simulink model "r_controller_system_integrated"  (R2024a)
settings: Solver=ode23tb  StartTime=0.0  StopTime=0.1  FixedStep=1e-5  MaxStep=1e-05  RelTol=1e-3
libraries: simulink x1
settings Model: Creator=PME406_01  LastModifiedBy=PME406_01

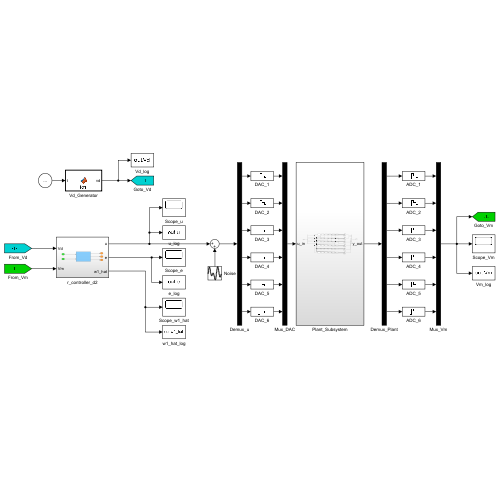
[thumbnail: Simulink's stored preview of the top-level diagram]
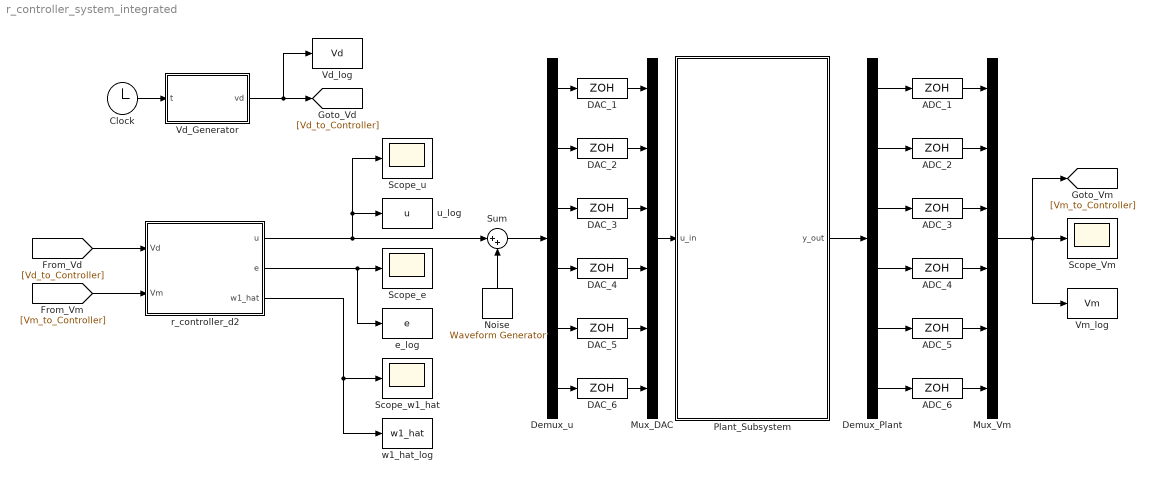
== system r_controller_system_integrated ==
  ADC_{1..6} (6 alike) : ZeroOrderHold  SampleTime=1e-05
  Clock : Clock
  DAC_{1..6} (6 alike) : ZeroOrderHold  SampleTime=1e-05
  Demux_Plant : Demux  Outputs=6
  Demux_u : Demux  Outputs=6
  Mux_DAC : Mux  Inputs=6
  Mux_Vm : Mux  Inputs=6
  Noise : simulink/Sources/Waveform Generator  OutMin=[]  OutMax=[]  OutDataTypeStr=double  SelectedSignal=1  BlockNames=MultiportSwitch_e3df3653d217406  SampleTime=0.1
  Plant_Subsystem : Subsystem
  Scope_Vm : Scope
  Scope_e : Scope
  Scope_u : Scope
  Scope_w1_hat : Scope
  Sum : Sum  Inputs=|++
  Vd_Generator : MATLAB Function  TreatAsAtomicUnit=on
  Vd_log : ToWorkspace  VariableName=Vd  SampleTime=-1
      settings: Save2DSignal=2-D array (concatenate along first dimension)
  Vm_log : ToWorkspace  VariableName=Vm  SampleTime=-1
      settings: Save2DSignal=2-D array (concatenate along first dimension)
  e_log : ToWorkspace  VariableName=e  SampleTime=-1
      settings: Save2DSignal=2-D array (concatenate along first dimension)
  r_controller_d2 : Subsystem
  u_log : ToWorkspace  VariableName=u  SampleTime=-1
      settings: Save2DSignal=2-D array (concatenate along first dimension)
  w1_hat_log : ToWorkspace  VariableName=w1_hat  SampleTime=-1
      settings: Save2DSignal=2-D array (concatenate along first dimension)
  wires:
  Vd_Generator/1(vd) -> Vd_log/1, [Vd_to_Controller]
  Clock/1 -> Vd_Generator/1(t)
  Mux_Vm/1 -> Vm_log/1, Scope_Vm/1, [Vm_to_Controller]
  ADC_6/1 -> Mux_Vm/6
  Demux_u/5 -> DAC_5/1
  DAC_4/1 -> Mux_DAC/4
  ADC_2/1 -> Mux_Vm/2
  Demux_u/6 -> DAC_6/1
  Sum/1 -> Demux_u/1
  ADC_4/1 -> Mux_Vm/4
  DAC_3/1 -> Mux_DAC/3
  r_controller_d2/1(u) -> Scope_u/1, u_log/1, Sum/1
  DAC_1/1 -> Mux_DAC/1
  DAC_2/1 -> Mux_DAC/2
  Demux_u/1 -> DAC_1/1
  Plant_Subsystem/1(y_out) -> Demux_Plant/1
  Demux_Plant/2 -> ADC_2/1
  Demux_Plant/5 -> ADC_5/1
  Noise/1 -> Sum/2
  ADC_3/1 -> Mux_Vm/3
  ADC_1/1 -> Mux_Vm/1
  r_controller_d2/3(w1_hat) -> w1_hat_log/1, Scope_w1_hat/1
  [Vm_to_Controller] -> r_controller_d2/2(Vm)
  Demux_Plant/4 -> ADC_4/1
  DAC_5/1 -> Mux_DAC/5
  Demux_u/3 -> DAC_3/1
  Demux_Plant/3 -> ADC_3/1
  Demux_Plant/1 -> ADC_1/1
  DAC_6/1 -> Mux_DAC/6
  Demux_u/4 -> DAC_4/1
  Mux_DAC/1 -> Plant_Subsystem/1(u_in)
  r_controller_d2/2(e) -> e_log/1, Scope_e/1
  Demux_u/2 -> DAC_2/1
  ADC_5/1 -> Mux_Vm/5
  Demux_Plant/6 -> ADC_6/1
  [Vd_to_Controller] -> r_controller_d2/1(Vd)

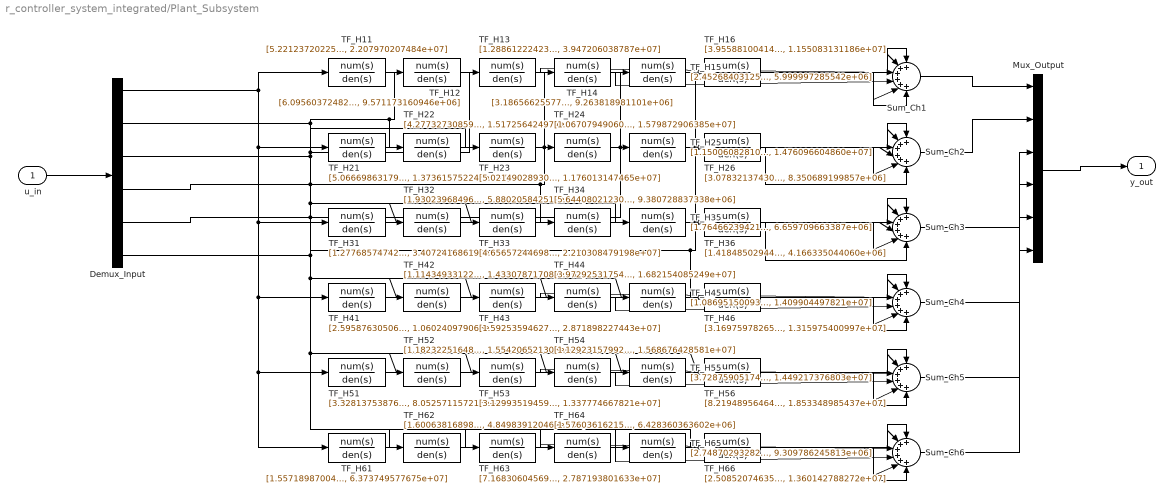
== system r_controller_system_integrated/Plant_Subsystem ==
  u_in : Inport
  Demux_Input : Demux  Outputs=6
  Mux_Output : Mux  Inputs=6
  Sum_Ch{1..6} (6 alike) : Sum  Inputs=++++++
  TF_H11 : TransferFcn  Numerator=[5.221237202258e+06]  Denominator=[1, 1.125476429798e+04, 2.207970207484e+07]
  TF_H12 : TransferFcn  Numerator=[6.095603724823e+04]  Denominator=[1, 1.615096196557e+03, 9.571173160946e+06]
  TF_H13 : TransferFcn  Numerator=[1.288612224236e+06]  Denominator=[1, 1.231137597589e+04, 3.947206038787e+07]
  TF_H14 : TransferFcn  Numerator=[3.186566255776e+05]  Denominator=[1, 7.765927137710e+03, 9.263818981101e+06]
  TF_H15 : TransferFcn  Numerator=[2.452684031253e+05]  Denominator=[1, 5.746401647961e+03, 5.999997285542e+06]
  TF_H16 : TransferFcn  Numerator=[3.955881004140e+05]  Denominator=[1, 3.580306515557e+03, 1.155083131186e+07]
  TF_H21 : TransferFcn  Numerator=[5.066698631790e+04]  Denominator=[1, 1.108261849372e+03, 1.373615752245e+07]
  TF_H22 : TransferFcn  Numerator=[4.277327308593e+06]  Denominator=[1, 1.003268373777e+04, 1.517256424974e+07]
  TF_H23 : TransferFcn  Numerator=[5.021490289304e+05]  Denominator=[1, 8.810895080316e+03, 1.176013147465e+07]
  TF_H24 : TransferFcn  Numerator=[1.067079490600e+06]  Denominator=[1, 1.135112820448e+04, 1.579872906385e+07]
  TF_H25 : TransferFcn  Numerator=[1.150060828107e+06]  Denominator=[1, 1.065992916636e+04, 1.476096604860e+07]
  TF_H26 : TransferFcn  Numerator=[3.078321374306e+05]  Denominator=[1, 6.847783968129e+03, 8.350689199857e+06]
  TF_H31 : TransferFcn  Numerator=[1.277685747428e+06]  Denominator=[1, 1.368269686933e+04, 3.407241686199e+07]
  TF_H32 : TransferFcn  Numerator=[1.930239684968e+05]  Denominator=[1, 4.560870597302e+03, 5.880205842512e+06]
  TF_H33 : TransferFcn  Numerator=[4.656572446985e+06]  Denominator=[1, 9.513164457161e+03, 2.210308479198e+07]
  TF_H34 : TransferFcn  Numerator=[5.644080212304e+04]  Denominator=[1, 1.954878812118e+03, 9.380728837338e+06]
  TF_H35 : TransferFcn  Numerator=[1.764662394212e+05]  Denominator=[1, 5.122349981324e+03, 6.659709663387e+06]
  TF_H36 : TransferFcn  Numerator=[1.418485029440e+05]  Denominator=[1, 1.438504147902e+03, 4.166335044060e+06]
  TF_H41 : TransferFcn  Numerator=[2.595876305066e+05]  Denominator=[1, 7.070165651413e+03, 1.060240979066e+07]
  TF_H42 : TransferFcn  Numerator=[1.114349331223e+06]  Denominator=[1, 9.846928206402e+03, 1.433078717084e+07]
  TF_H43 : TransferFcn  Numerator=[1.592535946272e+05]  Denominator=[1, 2.790294019501e+03, 2.871898227443e+07]
  TF_H44 : TransferFcn  Numerator=[3.972925317547e+06]  Denominator=[1, 1.159715140811e+04, 1.682154085249e+07]
  TF_H45 : TransferFcn  Numerator=[1.086951500933e+06]  Denominator=[1, 1.075231371220e+04, 1.409904497821e+07]
  TF_H46 : TransferFcn  Numerator=[3.169759782656e+05]  Denominator=[1, 8.067558736035e+03, 1.315975400997e+07]
  TF_H51 : TransferFcn  Numerator=[3.328137538766e+05]  Denominator=[1, 7.227274813518e+03, 8.052571157216e+06]
  TF_H52 : TransferFcn  Numerator=[1.182322516481e+06]  Denominator=[1, 1.030784744910e+04, 1.554206521303e+07]
  TF_H53 : TransferFcn  Numerator=[3.129935194599e+05]  Denominator=[1, 7.870328655037e+03, 1.337774667821e+07]
  TF_H54 : TransferFcn  Numerator=[1.129231579925e+06]  Denominator=[1, 1.104821595243e+04, 1.568676428581e+07]
  TF_H55 : TransferFcn  Numerator=[3.728759051745e+06]  Denominator=[1, 1.050075182774e+04, 1.449217376803e+07]
  TF_H56 : TransferFcn  Numerator=[8.219489564647e+04]  Denominator=[1, 1.407969854523e+03, 1.853348985437e+07]
  TF_H61 : TransferFcn  Numerator=[1.557189870041e+06]  Denominator=[1, 2.234640585923e+04, 6.373749577675e+07]
  TF_H62 : TransferFcn  Numerator=[1.600638168987e+05]  Denominator=[1, 3.864055922471e+03, 4.849839120469e+06]
  TF_H63 : TransferFcn  Numerator=[7.168306045699e+05]  Denominator=[1, 9.251556589809e+03, 2.787193801633e+07]
  TF_H64 : TransferFcn  Numerator=[1.576036162155e+05]  Denominator=[1, 4.743270970318e+03, 6.428360363602e+06]
  TF_H65 : TransferFcn  Numerator=[2.748702932822e+04]  Denominator=[1, 4.876033357949e+02, 9.309786245813e+06]
  TF_H66 : TransferFcn  Numerator=[2.508520746356e+06]  Denominator=[1, 5.985310903650e+03, 1.360142788272e+07]
  y_out : Outport
  wires:
  u_in/1 -> Demux_Input/1
  Demux_Input/1 -> TF_H11/1, TF_H51/1, TF_H61/1, TF_H41/1, TF_H31/1, TF_H21/1
  TF_H11/1 -> Sum_Ch1/1
  Demux_Input/2 -> TF_H12/1, TF_H22/1, TF_H52/1, TF_H62/1, TF_H42/1, TF_H32/1
  TF_H12/1 -> Sum_Ch1/2
  Demux_Input/3 -> TF_H13/1, TF_H23/1, TF_H53/1, TF_H63/1, TF_H43/1, TF_H33/1
  TF_H13/1 -> Sum_Ch1/3
  Demux_Input/4 -> TF_H54/1, TF_H64/1, TF_H44/1, TF_H14/1, TF_H24/1, TF_H34/1
  TF_H14/1 -> Sum_Ch1/4
  Demux_Input/5 -> TF_H55/1, TF_H65/1, TF_H45/1, TF_H15/1, TF_H25/1, TF_H35/1
  TF_H15/1 -> Sum_Ch1/5
  Demux_Input/6 -> TF_H16/1, TF_H26/1, TF_H36/1, TF_H46/1, TF_H56/1, TF_H66/1
  TF_H16/1 -> Sum_Ch1/6
  TF_H21/1 -> Sum_Ch2/1
  TF_H22/1 -> Sum_Ch2/2
  TF_H23/1 -> Sum_Ch2/3
  TF_H24/1 -> Sum_Ch2/4
  TF_H25/1 -> Sum_Ch2/5
  TF_H26/1 -> Sum_Ch2/6
  TF_H31/1 -> Sum_Ch3/1
  TF_H32/1 -> Sum_Ch3/2
  TF_H33/1 -> Sum_Ch3/3
  TF_H34/1 -> Sum_Ch3/4
  TF_H35/1 -> Sum_Ch3/5
  TF_H36/1 -> Sum_Ch3/6
  TF_H41/1 -> Sum_Ch4/1
  TF_H42/1 -> Sum_Ch4/2
  TF_H43/1 -> Sum_Ch4/3
  TF_H44/1 -> Sum_Ch4/4
  TF_H45/1 -> Sum_Ch4/5
  TF_H46/1 -> Sum_Ch4/6
  TF_H51/1 -> Sum_Ch5/1
  TF_H52/1 -> Sum_Ch5/2
  TF_H53/1 -> Sum_Ch5/3
  TF_H54/1 -> Sum_Ch5/4
  TF_H55/1 -> Sum_Ch5/5
  TF_H56/1 -> Sum_Ch5/6
  TF_H61/1 -> Sum_Ch6/1
  TF_H62/1 -> Sum_Ch6/2
  TF_H63/1 -> Sum_Ch6/3
  TF_H64/1 -> Sum_Ch6/4
  TF_H65/1 -> Sum_Ch6/5
  TF_H66/1 -> Sum_Ch6/6
  Sum_Ch1/1 -> Mux_Output/1
  Sum_Ch2/1 -> Mux_Output/2
  Sum_Ch3/1 -> Mux_Output/3
  Sum_Ch4/1 -> Mux_Output/4
  Sum_Ch5/1 -> Mux_Output/5
  Sum_Ch6/1 -> Mux_Output/6
  Mux_Output/1 -> y_out/1

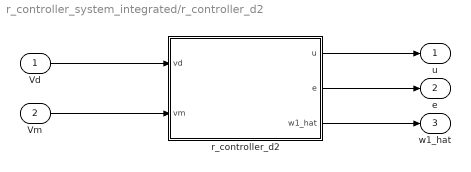
== system r_controller_system_integrated/r_controller_d2 ==
  Vd : Inport
  Vm : Inport  Port=2
  r_controller_d2 : MATLAB Function  TreatAsAtomicUnit=on
  u : Outport
  e : Outport  Port=2
  w1_hat : Outport  Port=3
  wires:
  r_controller_d2/3(w1_hat) -> w1_hat/1
  r_controller_d2/2(e) -> e/1
  Vm/1 -> r_controller_d2/2(vm)
  Vd/1 -> r_controller_d2/1(vd)
  r_controller_d2/1(u) -> u/1

== matlab function r_controller_system_integrated/r_controller_d2/r_controller_d2 ==
  settings: updateMethod=DISCRETE  sampleTime=1e-5
  data: vd input size=6; u output size=6; vm input size=6; e output size=6; w1_hat output size=6
function [u, e, w1_hat] = r_controller_function_d2(vd, vm)
    % R Controller with d=2 Preview (Flux_Control_R_newmodel.pdf Page 1)
    %
    % 完全平移時序方案：所有估測器公式從 k+1 平移到 k
    % 輸入：
    %   vd - 參考電壓向量 [6×1]（需要外部提供 3 步 preview）
    %   vm - 測量電壓向量 [6×1]
    % 輸出：
    %   u      - 控制輸入向量 [6×1]
    %   e      - 追蹤誤差向量 [6×1]（定義為 δv[k]）
    %   w1_hat - 干擾估測向量 [6×1]（用於監測干擾大小）
    %
    % Author: Claude Code
    % Date: 2025-10-16
    % Reference: Flux_Control_R_newmodel.pdf Page 1

    % ═══════════════════════════════════════════════════════════════════
    %                    SECTION 1: 參數定義
    % ═══════════════════════════════════════════════════════════════════

    % --- 系統模型參數 (from H(z^-1)) ---
    k_o = 5.6695e-4;              % k_o from H(z^-1)
    b = 0.9782;                   % b from H(z^-1)
    a1 = 1.934848;                % a1
    a2 = -0.935970;               % a2

    % --- B 矩陣 (6×6) ---
    B = [0.2365  -0.0064  -0.0327  -0.0344  -0.0408  -0.0343;
        -0.0037   0.2818  -0.0427  -0.0675  -0.0779  -0.0368;
        -0.0375  -0.0328   0.2108  -0.0060  -0.0265  -0.0341;
        -0.0245  -0.0777  -0.0056   0.2361  -0.0770  -0.0241;
        -0.0413  -0.0760  -0.0234  -0.0720   0.2572  -0.0045;
        -0.0244  -0.0330  -0.0257  -0.0245  -0.0030   0.1845];

    % --- B 反矩陣 ---
    B_inv = inv(B);

    % --- 控制參數 ---
    lambda_c = 0.8179;            % λc - 控制器特徵值
    lambda_e = 0.3659;            % λe - 估測器特徵值
    beta = lambda_c^2;            % β

    % --- 派生參數 ---
    kc = (1 - lambda_c) / (1 + b);
    bc = b * kc;
    ku = kc / k_o;

    % --- 估測器增益 ---
    % ℓ1
    l_1 = lambda_c + (1 + beta) - 3*lambda_e;

    % ℓ2
    l_2 = (b*(lambda_e - 1)^3 - beta*(b + 1)*(beta^2 - 3*beta*lambda_e + beta + 3*lambda_e^2 - 3*lambda_e + 1)) / ...
          (kc * (b + 1) * (b + beta));

    % ℓ3
    l_3 = (-(b + beta)*(beta^2 - 3*beta*lambda_e + beta + 3*lambda_e^2 - 3*lambda_e + 1) - lambda_e^3) / ...
          (kc * (b + 1) * (b + beta));

    % ═══════════════════════════════════════════════════════════════════
    %              SECTION 2: Persistent 變數聲明與初始化
    % ═══════════════════════════════════════════════════════════════════

    % --- VD Buffer (d=2 需要 4 層) ---
    persistent vd_buffer          % vd buffer: [vd[k]; vd[k+1]; vd[k+2]; vd[k+3]]

    % --- VF 預濾波器歷史 ---
    persistent vf                 % vf[k] - 當前時刻
    persistent vf_k1              % vf[k-1] - 過去 1 步

    % --- 增量歷史 ---
    persistent delta_vf_k1        % δvf[k-1]
    persistent delta_v_k1         % δv[k-1]

    % --- 估測器狀態歷史 ---
    persistent delta_v_hat_k1     % δv̂[k-1]
    persistent w1_hat_k1          % ŵ1[k-1]
    persistent w2_hat_k1          % ŵ2[k-1]

    % --- 控制律歷史 ---
    persistent uc_k1              % uc[k-1]
    persistent uc_k2              % uc[k-2]
    persistent delta_vc_k1        % δvc[k-1]
    persistent delta_vc_k2        % δvc[k-2]

    % --- 初始化標誌 ---
    persistent initialized

    if isempty(initialized)
        initialized = true;

        % Buffer 初始化（4 層：k, k+1, k+2, k+3）
        vd_buffer = zeros(4, 6);  % Row 1: vd[k], Row 2: vd[k+1], Row 3: vd[k+2], Row 4: vd[k+3]

        % VF 濾波器初始化
        vf = zeros(6, 1);
        vf_k1 = zeros(6, 1);

        % 增量初始化
        delta_vf_k1 = zeros(6, 1);
        delta_v_k1 = zeros(6, 1);

        % 估測器初始化
        delta_v_hat_k1 = zeros(6, 1);
        w1_hat_k1 = zeros(6, 1);
        w2_hat_k1 = zeros(6, 1);

        % 控制律初始化
        uc_k1 = zeros(6, 1);
        uc_k2 = zeros(6, 1);
        delta_vc_k1 = zeros(6, 1);
        delta_vc_k2 = zeros(6, 1);
    end

    % ═══════════════════════════════════════════════════════════════════
    %                SECTION 3: VD Buffer 管理 (d=2)
    % ═══════════════════════════════════════════════════════════════════

    % Buffer 更新：vd[k] <- vd[k+1] <- vd[k+2] <- vd[k+3] <- new input
    vd_buffer(1, :) = vd_buffer(2, :);  % vd[k] = old vd[k+1]
    vd_buffer(2, :) = vd_buffer(3, :);  % vd[k+1] = old vd[k+2]
    vd_buffer(3, :) = vd_buffer(4, :);  % vd[k+2] = old vd[k+3]
    vd_buffer(4, :) = vd';              % vd[k+3] = new input (假設外部已 preview)

    % 提取各時刻的 vd（轉置為列向量）
    vd_k        = vd_buffer(1, :)';  % vd[k] - 當前時刻
    vd_k_plus1  = vd_buffer(2, :)';  % vd[k+1] - preview 1 步
    vd_k_plus2  = vd_buffer(3, :)';  % vd[k+2] - preview 2 步
    vd_k_plus3  = vd_buffer(4, :)';  % vd[k+3] - preview 3 步

    % ═══════════════════════════════════════════════════════════════════
    %             SECTION 4: VF 預濾波器計算 (PDF Step 1, d=2)
    % ═══════════════════════════════════════════════════════════════════

    % vf[k+1] = 1/((1-λc)(1+b)) {b·vd[k+3] + (1-b·λc)·vd[k+2] - λc·vd[k+1]}
    vf_next = (1 / ((1 - lambda_c) * (1 + b))) * ...
              (b * vd_k_plus3 + (1 - b*lambda_c) * vd_k_plus2 - lambda_c * vd_k_plus1);

    % ═══════════════════════════════════════════════════════════════════
    %              SECTION 5: 增量計算 (PDF Step 2)
    % ═══════════════════════════════════════════════════════════════════

    % δvf[k] = vf[k+1] - (1-bc)·vf[k] - bc·vf[k-1]
    delta_vf = vf_next - (1 - bc)*vf - bc*vf_k1;

    % δv[k] = vf[k] - vm[k]
    delta_v = vf - vm;

    % ═══════════════════════════════════════════════════════════════════
    %          SECTION 6: 估測器狀態更新 (PDF Step 3, 完全平移)
    % ═══════════════════════════════════════════════════════════════════

    % 誤差項（使用 k-1 時刻的資訊）
    error_term = delta_v_k1 - delta_v_hat_k1;

    % δv̂[k] = λc·δv̂[k-1] + δvf[k-1] + ℓ1{δv[k-1] - δv̂[k-1]}
    delta_v_hat = lambda_c * delta_v_hat_k1 + delta_vf_k1 + l_1 * error_term;

    % ŵ1[k] = (1+β)·ŵ1[k-1] - β·ŵ2[k-1] + ℓ2{δv[k-1] - δv̂[k-1]}
    w1_hat = (1 + beta) * w1_hat_k1 - beta * w2_hat_k1 + l_2 * error_term;

    % ŵ2[k] = ŵ1[k-1] + ℓ3{δv[k-1] - δv̂[k-1]}
    w2_hat = w1_hat_k1 + l_3 * error_term;

    % ═══════════════════════════════════════════════════════════════════
    %                  SECTION 7: 控制律計算 (PDF Step 4)
    % ═══════════════════════════════════════════════════════════════════

    % δvc[k] = δv[k] - ŵ1[k]
    delta_vc = delta_v - w1_hat;

    % uc[k] = (1-bc)·uc[k-1] - bc·uc[k-2] + ku·{δvc[k] - a1·δvc[k-1] - a2·δvc[k-2]}
    uc = (1 - bc) * uc_k1 - bc * uc_k2 + ...
         ku * (delta_vc - a1 * delta_vc_k1 - a2 * delta_vc_k2);

    % u[k] = B^(-1)·uc[k]
    u = B_inv * uc;

    % 輸出誤差（定義為 δv[k]）
    e = delta_v;

    % ═══════════════════════════════════════════════════════════════════
    %               SECTION 8: 歷史變數更新（為下一時刻準備）
    % ═══════════════════════════════════════════════════════════════════

    % VF 濾波器歷史更新
    vf_k1 = vf;        % vf[k-1] ← vf[k]
    vf = vf_next;      % vf[k] ← vf[k+1]

    % 增量歷史更新
    delta_vf_k1 = delta_vf;  % δvf[k-1] ← δvf[k]
    delta_v_k1 = delta_v;    % δv[k-1] ← δv[k]

    % 估測器歷史更新
    delta_v_hat_k1 = delta_v_hat;  % δv̂[k-1] ← δv̂[k]
    w1_hat_k1 = w1_hat;            % ŵ1[k-1] ← ŵ1[k]
    w2_hat_k1 = w2_hat;            % ŵ2[k-1] ← ŵ2[k]

    % 控制律歷史更新
    uc_k2 = uc_k1;              % uc[k-2] ← uc[k-1]
    uc_k1 = uc;                 % uc[k-1] ← uc[k]
    delta_vc_k2 = delta_vc_k1;  % δvc[k-2] ← δvc[k-1]
    delta_vc_k1 = delta_vc;     % δvc[k-1] ← δvc[k]
end

== matlab function r_controller_system_integrated/Vd_Generator ==
  settings: updateMethod=DISCRETE  sampleTime=1e-5
  data: t input; vd output size=6
function vd = fcn(t)
    % Vd Generator with Preview - Workspace Version
    % 從 workspace 讀取 vd_params 來動態配置信號參數
    % Preview: 使用 t + Ts 來實現一個採樣週期的時間超前
    
    % 宣告外部函數（用於從 workspace 讀取）
    coder.extrinsic('evalin');
    
    % 固定參數
    Ts = 1e-5;  % 採樣週期 (100 kHz)
    
    % 預設值（如果 workspace 沒有 vd_params）
    channel = 1;
    amplitude = 0.1;
    frequency = 60;
    
    % 從 workspace 讀取參數
    if coder.target('MATLAB')
        try
            params = evalin('base', 'vd_params');
            channel = params.channel;
            amplitude = params.amplitude;
            frequency = params.frequency;
        catch
            % 使用預設值（workspace 中沒有 vd_params）
        end
    end
    
    % ★ Preview 機制：使用未來時間點
    t_future = t + Ts;
    
    % 輸出 6 通道向量
    vd = zeros(6, 1);
    vd(channel) = amplitude * sin(2*pi*frequency*t_future);
end
